simulink model "SpringMassDamper"  (R2018b)
settings: Solver=VariableStepAuto  StartTime=0.0  StopTime=10.0  RelTol=1e-3
settings Model: Creator=Notebook  LastModifiedBy=Notebook

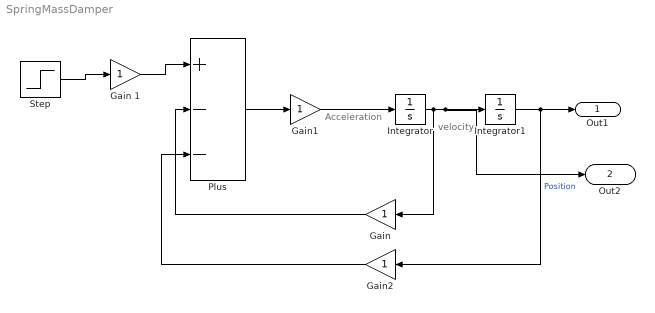
== system SpringMassDamper ==
  note: velocity
  note: Acceleration
  Gain : Gain
  Gain 1 : Gain
  Gain1 : Gain
  Gain2 : Gain
  Integrator : Integrator
  Integrator1 : Integrator
  Plus : Sum  Inputs=+--
  Step : Step  SampleTime=0
  Out1 : Outport  SignalName=position
  Out2 : Outport  Port=2
  wires:
  Step/1 -> Gain 1/1
  Gain 1/1 -> Plus/1
  Plus/1 -> Gain1/1
  Gain1/1 -> Integrator/1
  Integrator/1 -> Integrator1/1, Out2/1, Gain/1
  Integrator1/1 -> Gain2/1, Out1/1  "Position"
  Gain/1 -> Plus/2
  Gain2/1 -> Plus/3
